simulink model "Distance_final_UG_spring2022"  (R2020b)
settings: Solver=ode3  StartTime=0.0  StopTime=0.2  FixedStep=1e-6  RelTol=1e-3
InitFcn:
  | Ts=1/1200; Ts_Power=1e-6;
StartFcn:
  | Ts=1/1200;Ts_Power=1e-6;
libraries: powerlib x11, powerlib_meascontrol x3, simulink x1
(part 2 of 2)

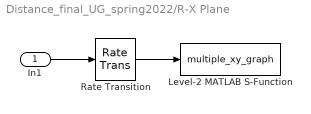
== system Distance_final_UG_spring2022/R-X Plane ==
  In1 : Inport
  Level-2 MATLAB S-Function : M-S-Function  FunctionName=multiple_xy_graph  Parameters=number_of_trajectories,axis_limits
  Rate Transition : RateTransition  OutPortSampleTime=sample_time
  wires:
  In1/1 -> Rate Transition/1
  Rate Transition/1 -> Level-2 MATLAB S-Function/1

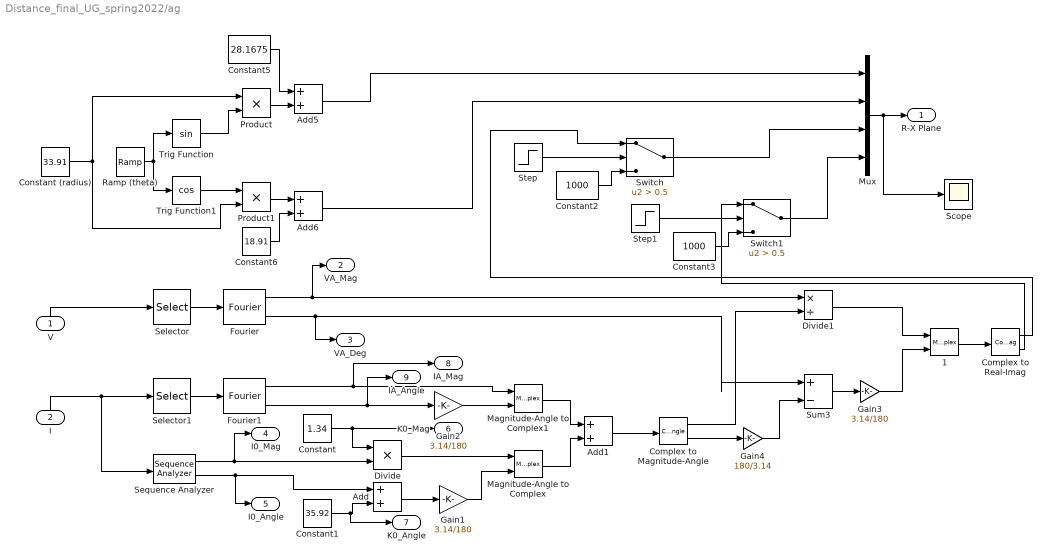
== system Distance_final_UG_spring2022/ag ==
  V : Inport
  I : Inport  Port=2
  1 : MagnitudeAngleToComplex
  Add{,1,5..6} (4 alike) : Sum
  Complex to Magnitude-Angle : ComplexToMagnitudeAngle
  Complex to Real-Imag : ComplexToRealImag
  Constant : Constant  Value=1.34
  Constant (radius) : Constant  Value=33.91
  Constant1 : Constant  Value=35.92
  Constant2 : Constant  Value=1000
  Constant3 : Constant  Value=1000
  Constant5 : Constant  Value=28.1675
  Constant6 : Constant  Value=18.91
  Divide : Product  Inputs=**
  Divide1 : Product  Inputs=*/
  Fourier : powerlib_meascontrol/Measurements/Fourier  Freq=60  n=1  InInit=[0, 0]  Ts=Ts_Power
  Fourier1 : powerlib_meascontrol/Measurements/Fourier  Freq=60  n=1  InInit=[0, 0]  Ts=Ts_Power
  Gain1 : Gain  Gain=3.14/180
  Gain2 : Gain  Gain=3.14/180
  Gain3 : Gain  Gain=3.14/180
  Gain4 : Gain  Gain=180/3.14
  Magnitude-Angle to Complex : MagnitudeAngleToComplex
  Magnitude-Angle to Complex1 : MagnitudeAngleToComplex
  Mux : Mux
  Product : Product  RndMeth=Zero
  Product1 : Product  RndMeth=Zero
  Ramp (theta) : simulink/Sources/Ramp  slope=33.875  start=0  InitialOutput=0  VectorParams1D=off
  Scope : Scope
  Selector : Selector  InputPortWidth=3  IndexOptions=Index vector (dialog)  Indices=[1]  OutputSizes=1
  Selector1 : Selector  InputPortWidth=3  IndexOptions=Index vector (dialog)  Indices=[1]  OutputSizes=1
  Sequence Analyzer : powerlib_meascontrol/Measurements/Sequence Analyzer  Freq=60  n=1  seq=Zero  InInit=[1, 0]  Ts=Ts_Power
      settings: SourceProductBaseCode=PS
  Step : Step  Time=0.02  SampleTime=0
  Step1 : Step  Time=0.02  SampleTime=0
  Sum3 : Sum  Inputs=|+-
  Switch : Switch  Criteria=u2 > Threshold  Threshold=0.5
  Switch1 : Switch  Criteria=u2 > Threshold  Threshold=0.5
  Trig Function : Trigonometry
  Trig Function1 : Trigonometry  Operator=cos
  R-X Plane : Outport  VectorParamsAs1DForOutWhenUnconnected=off
  VA_Mag : Outport  Port=2  VectorParamsAs1DForOutWhenUnconnected=off
  VA_Deg : Outport  Port=3  VectorParamsAs1DForOutWhenUnconnected=off
  I0_Mag : Outport  Port=4  VectorParamsAs1DForOutWhenUnconnected=off
  I0_Angle : Outport  Port=5  VectorParamsAs1DForOutWhenUnconnected=off
  K0_Mag : Outport  Port=6  VectorParamsAs1DForOutWhenUnconnected=off
  K0_Angle : Outport  Port=7  VectorParamsAs1DForOutWhenUnconnected=off
  IA_Mag : Outport  Port=8  VectorParamsAs1DForOutWhenUnconnected=off
  IA_Angle : Outport  Port=9  VectorParamsAs1DForOutWhenUnconnected=off
  wires:
  Fourier1/2 -> IA_Angle/1, Gain2/1
  Sequence Analyzer/2 -> I0_Angle/1, Add/1
  Add/1 -> Gain1/1
  Magnitude-Angle to Complex1/1 -> Add1/1
  Magnitude-Angle to Complex/1 -> Add1/2
  Selector1/1 -> Fourier1/1
  Gain4/1 -> Sum3/2
  Selector/1 -> Fourier/1
  Complex to Magnitude-Angle/1 -> Divide1/2
  Add1/1 -> Complex to Magnitude-Angle/1
  Fourier/2 -> VA_Deg/1, Sum3/1
  Sequence Analyzer/1 -> I0_Mag/1, Divide/2
  Fourier1/1 -> IA_Mag/1, Magnitude-Angle to Complex1/1
  1/1 -> Complex to Real-Imag/1
  Sum3/1 -> Gain3/1
  Divide1/1 -> 1/1
  Gain3/1 -> 1/2
  Fourier/1 -> VA_Mag/1, Divide1/1
  Gain2/1 -> Magnitude-Angle to Complex1/2
  Divide/1 -> Magnitude-Angle to Complex/1
  Gain1/1 -> Magnitude-Angle to Complex/2
  Complex to Magnitude-Angle/2 -> Gain4/1
  Constant/1 -> K0_Mag/1, Divide/1
  Constant1/1 -> K0_Angle/1, Add/2
  V/1 -> Selector/1
  I/1 -> Selector1/1, Sequence Analyzer/1
  Trig Function1/1 -> Product1/1
  Ramp (theta)/1 -> Trig Function/1, Trig Function1/1
  Constant (radius)/1 -> Product/1, Product1/2
  Trig Function/1 -> Product/2
  Product/1 -> Add5/2
  Constant5/1 -> Add5/1
  Product1/1 -> Add6/1
  Constant6/1 -> Add6/2
  Add6/1 -> Mux/2
  Add5/1 -> Mux/1
  Mux/1 -> Scope/1, R-X Plane/1
  Constant2/1 -> Switch/3
  Step/1 -> Switch/2
  Complex to Real-Imag/1 -> Switch/1
  Step1/1 -> Switch1/2
  Constant3/1 -> Switch1/3
  Complex to Real-Imag/2 -> Switch1/1
  Switch/1 -> Mux/3
  Switch1/1 -> Mux/4
